simulink model "TrafficLight_StateFlow"  (R2024a)
settings: Solver=FixedStepDiscrete  StartTime=0.0  StopTime=inf  RelTol=1e-3  EnableMultiTasking=on
libraries: arduinolib x4, simulink x1
settings Model: ExtModeTrigDuration=2  Creator=VICTUS  LastModifiedBy=VICTUS
settings SolverCC: AutoInsertRateTranBlk=on
settings OptimizationCC: EnhancedBackFolding=on  PassReuseOutputArgsAs=Individual arguments  ZeroExternalMemoryAtStartup=off  ZeroInternalMemoryAtStartup=off  MaxStackSize=64  OptimizeBlockOrder=speed  DifferentSizesBufferReuse=on  OptimizationCustomize=off  EfficientTunableParamExpr=on
settings DebuggingCC: ParameterTunabilityLossMsg=error
settings HardwareCC: ProdBitPerPointer=32  ProdBitPerSizeT=32  ProdBitPerPtrDiffT=32  ProdLargestAtomicInteger=Long  ProdLargestAtomicFloat=Double  ProdWordSize=32  ProdHWDeviceType=ARM Compatible->ARM Cortex
settings SFSimCC: MATLABDynamicMemAlloc=off
settings RTWCC: Description=Embedded Coder  SystemTargetFile=ert.tlc  HardwareBoard=ESP32-WROOM(Arduino Compatible)  TLCOptions="-aInlineSetEventsForThisBaseRateFcn=TLC_FALSE -aSuppressMultiTaskScheduler=TLC_FALSE  -aRateBasedStepFcn=0"  TemplateMakefile=ert_default_tmf  Toolchain=ESP32  BuildConfiguration=Faster Runs
settings CodeAppCC: ForceParamTrailComments=on  IgnoreCustomStorageClasses=off  OperatorAnnotations=on  SimulinkDataObjDesc=on  SFDataObjDesc=on  InsertBlockDesc=on
settings ERTTargetCC: SupportContinuousTime=on  SupportVariableSizeSignals=on  ExtModeTransport=3  ExtModeStaticAlloc=on  ExtModeAutomaticAllocSize=off  ExtModeStaticAllocSize=65536  ExtModeMexFile=ext_xcp  ExtModeIntrfLevel=Level2 - Open

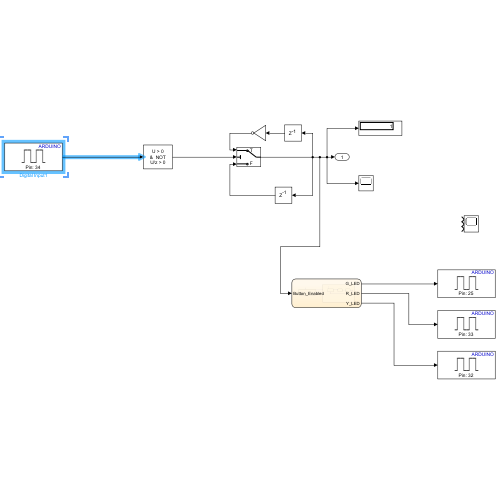
[thumbnail: Simulink's stored preview of the top-level diagram]
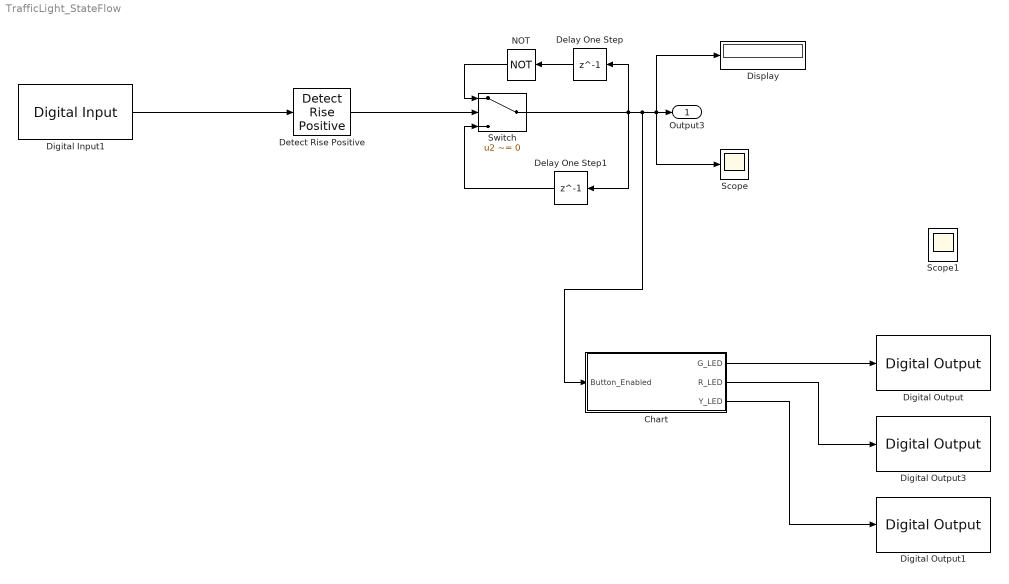
== system TrafficLight_StateFlow ==
  Chart : Stateflow chart  TreatAsAtomicUnit=on
  Delay One Step : Delay  DelayLength=1
  Delay One Step1 : Delay  DelayLength=1
  Detect Rise Positive : simulink/Logic and Bit Operations/Detect Rise Positive  vinit=0  OutDataTypeStr=boolean
  Digital Input1 : arduinolib/Digital Input  pinNumber=34  mode=Default  Direction=input  SampleTime=-1  blockPlatform=arduino
  Digital Output : arduinolib/Digital Output  pinNumber=25  Direction=output  blockPlatform=arduino
  Digital Output1 : arduinolib/Digital Output  pinNumber=32  Direction=output  blockPlatform=arduino
  Digital Output3 : arduinolib/Digital Output  pinNumber=33  Direction=output  blockPlatform=arduino
  Display : Display
  NOT : Logic  Operator=NOT  IconShape=distinctive  AllPortsSameDT=off  OutDataTypeStr=boolean
  Scope : Scope
  Scope1 : Scope  NumInputPorts=3
  Switch : Switch  Criteria=u2 ~= 0  SaturateOnIntegerOverflow=off  InputSameDT=off
  Output3 : Outport
  wires:
  Delay One Step/1 -> NOT/1
  Detect Rise Positive/1 -> Switch/2
  Switch/1 -> Scope/1, Display/1, Output3/1, Chart/1(Button_Enabled), Delay One Step/1, Delay One Step1/1
  Delay One Step1/1 -> Switch/3
  NOT/1 -> Switch/1
  Digital Input1/1 -> Detect Rise Positive/1
  Chart/1(G_LED) -> Digital Output/1
  Chart/3(Y_LED) -> Digital Output1/1
  Chart/2(R_LED) -> Digital Output3/1

== stateflow chart TrafficLight_StateFlow/Chart ==
  settings: executeAtInitialization=1
  state TrafficLight
    state Green
      du:
      G_LED = 1;
      Y_LED = 0;
      R_LED = 0;
    state Yellow
      du:
      G_LED = 0;
      Y_LED = 1;
      R_LED = 0;
    state Red
      du:
      G_LED = 0;
      Y_LED = 0;
      R_LED = 1;
    (default) -> Green
    Green -> Yellow : after(10,sec)
    Red -> (junction 32)
    Yellow -> Red : after(10,sec)
    (junction 32) -> (junction 34)
    (junction 36) -> Green
    (junction 34) -> (junction 36) : after(10,sec)
  state Crossing
    du:
    G_LED = 0;
    Y_LED = 0;
    R_LED = 0;
  (default) -> Crossing
  Crossing -> TrafficLight : [Button_Enabled == 1]
  TrafficLight -> Crossing : [Button_Enabled == 0]
  data: G_LED output; R_LED output; Y_LED output; Button_Enabled input double
